simulink model "RADIAL_BOOST"  (R2020b)
settings: Solver=ode4  StartTime=0.0  StopTime=10000  FixedStep=Dt  RelTol=1e-3
values from neighbouring files (symbols this model uses):
  alpha = 0.01    [INPUTS_GRUPPO20.m]
  dt_RB = m_c0_RB*(dv_RB)/F_thr    [INPUTS_GRUPPO20.m]
  e_ss = 0.02    [INPUTS_GRUPPO20.m]
  enable_drag = 1    [INPUTS_GRUPPO20.m]
  enable_J2 = 1    [INPUTS_GRUPPO20.m]
  enable_Mgrav = 1    [INPUTS_GRUPPO20.m]
  enable_PD = 1    [INPUTS_GRUPPO20.m]
  enable_SMC = 0    [INPUTS_GRUPPO20.m]
  F_D = -1/2*rho*CD*A*Vx^2    (= -3.88125057814e-05)    [INPUTS_GRUPPO20.m]
  F_thr = n*Tmax    (= 2)    [INPUTS_GRUPPO20.m]
  FJ2 = -3*J2*m_c0*mu*r_E^2/(2*r^4)    (= -0.00149705073945)    [INPUTS_GRUPPO20.m]
  gmax = 0.005    [INPUTS_GRUPPO20.m]
  INV_ZZZ = pinv(ZZZ)    [INPUTS_GRUPPO20.m]
  invJ = inv(J)    [INPUTS_GRUPPO20.m]
  Isp1 = 220    [INPUTS_GRUPPO20.m]
  J = J0    [INPUTS_GRUPPO20.m]
  kd = d*eye(3)    [INPUTS_GRUPPO20.m]
  kf = U_max/edb    (= 10)    [INPUTS_GRUPPO20.m]
  kp1 = k*eye(3)    [INPUTS_GRUPPO20.m]
  Kr = 1    [INPUTS_GRUPPO20.m]
  lambda = 0.03    [INPUTS_GRUPPO20.m]
  m_c0_RB = m_H(end)    [INPUTS_GRUPPO20.m]
  omega = (mu/r^3)^0.5    (= 0.00113136572666)    [INPUTS_GRUPPO20.m]
  p_RW = 1    [INPUTS_GRUPPO20.m]
  Pos0 = Pos_RB(end,:)'    [INPUTS_GRUPPO20.m]
  q0_0 = Q_RB(end,1)'    [INPUTS_GRUPPO20.m]
  q_des = [1 0 0 0]'    [INPUTS_GRUPPO20.m]
  qv_0 = Q_RB(end,2:4)'    [INPUTS_GRUPPO20.m]
  tau = -deltaton/log((1-(U_on-U_off)/kf))    [INPUTS_GRUPPO20.m]
  tau_RW = 1.5645e-2    (= 0.015645)    [INPUTS_GRUPPO20.m]
  U_max = 2    [INPUTS_GRUPPO20.m]
  U_off = 0.29    [INPUTS_GRUPPO20.m]
  U_on = 1    [INPUTS_GRUPPO20.m]
  Vel0 = Vel_RB(end,:)'    [INPUTS_GRUPPO20.m]
  wb_0 = wb_RB(end,:)'    [INPUTS_GRUPPO20.m]
  ZZZ = [cos(B)    0      -cos(B)    0 ... (first row only)    [INPUTS_GRUPPO20.m]
undefined symbols (not defined in the file or in its folder): DiscIntNeverNeededParam, magnitude
libraries: vrlib x3, aerolibutil x1, sharedtransform x1
settings Model: Creator=andre  LastModifiedBy=andre

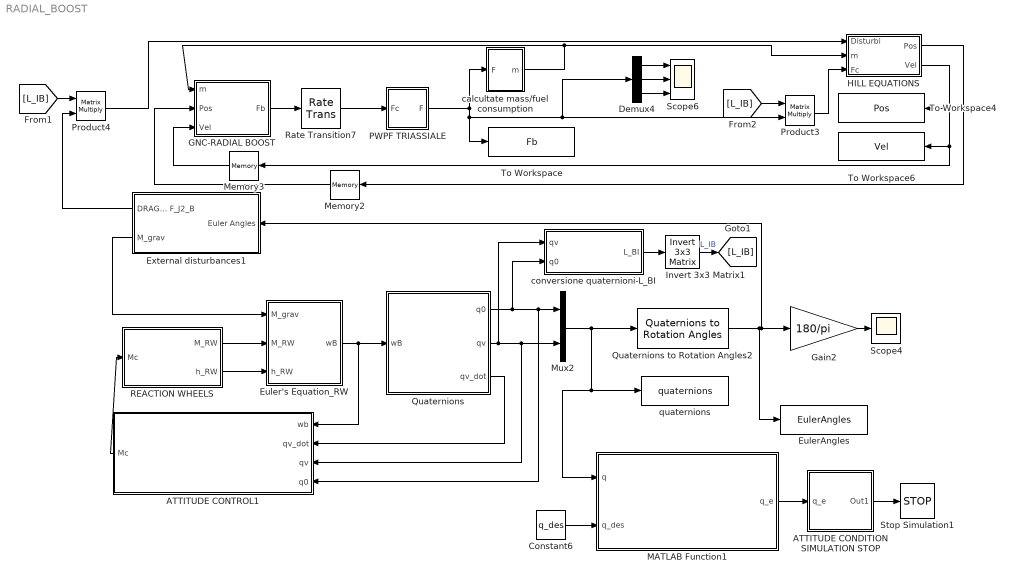
== system RADIAL_BOOST ==
  ATTITUDE CONDITION SIMULATION STOP : Subsystem
  ATTITUDE CONTROL1 : Subsystem
  Constant6 : Constant  Value=q_des
  Demux4 : Demux  Outputs=3
  Euler's Equation_RW : Subsystem
  EulerAngles : ToWorkspace  VariableName=EulerAngles  SampleTime=-1
  External disturbances1 : Subsystem
  GNC-RADIAL BOOST : Subsystem
  Gain2 : Gain  Gain=180/pi
  HILL EQUATIONS : Subsystem
  Invert 3x3 Matrix1 : aerolibutil/Invert  3x3 Matrix
  MATLAB Function1 : MATLAB Function  TreatAsAtomicUnit=on
  Memory2 : Memory  InitialCondition=Pos0
  Memory3 : Memory  InitialCondition=Vel0
  Mux2 : Mux  Inputs=2
  PWPF TRIASSIALE : Subsystem
  Product3 : Product  Multiplication=Matrix(*)
  Product4 : Product  Multiplication=Matrix(*)
  Quaternions : Subsystem
  Quaternions to Rotation Angles2 : sharedtransform/Quaternions to Rotation Angles  rotationOrder=ZYX  aMode=aMode
      settings: SourceProductBaseCode=AE,PW,MT,UV,VE,VP
  REACTION WHEELS : Subsystem
  Rate Transition7 : RateTransition  OutPortSampleTime=Dt
  Scope4 : Scope
  Scope6 : Scope  NumInputPorts=3
  Stop Simulation1 : Stop
  To Workspace : ToWorkspace  VariableName=Fb  SampleTime=-1
  To Workspace4 : ToWorkspace  VariableName=Pos  SampleTime=-1
      settings: Save2DSignal=2-D array (concatenate along first dimension)
  To Workspace6 : ToWorkspace  VariableName=Vel  SampleTime=-1
      settings: Save2DSignal=2-D array (concatenate along first dimension)
  calcultate mass/fuel consumption : Subsystem
  conversione quaternioni-L_BI : Subsystem
  quaternions : ToWorkspace  VariableName=quaternions  SampleTime=-1
  wires:
  Demux4/1 -> Scope6/1
  calcultate mass/fuel consumption/1(m) -> GNC-RADIAL BOOST/1(m), HILL EQUATIONS/2(m)
  [L_IB] -> Product3/1
  conversione quaternioni-L_BI/1(L_BI) -> Invert 3x3 Matrix1/1
  Memory3/1 -> GNC-RADIAL BOOST/3(Vel)
  Gain2/1 -> Scope4/1
  External disturbances1/2(M_grav) -> Euler's Equation_RW/1(M_grav)
  Quaternions/3(qv_dot) -> ATTITUDE CONTROL1/2(qv_dot)
  GNC-RADIAL BOOST/1(Fb) -> Rate Transition7/1
  Rate Transition7/1 -> PWPF TRIASSIALE/1(Fc)
  Quaternions to Rotation Angles2/1 -> Gain2/1, External disturbances1/1(Euler Angles), EulerAngles/1
  [L_IB] -> Product4/1
  HILL EQUATIONS/2(Vel) -> Memory3/1, To Workspace6/1
  PWPF TRIASSIALE/1(F) -> Demux4/1, Product3/2, To Workspace/1, calcultate mass/fuel consumption/1(F)
  REACTION WHEELS/2("h_RW ") -> Euler's Equation_RW/3(h_RW)
  Invert 3x3 Matrix1/1 -> [L_IB]  "L_IB"
  Demux4/3 -> Scope6/3
  Product3/1 -> HILL EQUATIONS/3(Fc)
  Product4/1 -> HILL EQUATIONS/1(Disturbi)
  Memory2/1 -> GNC-RADIAL BOOST/2(Pos)
  Quaternions/1(q0) -> ATTITUDE CONTROL1/4(q0), Mux2/1, conversione quaternioni-L_BI/2(q0)
  Constant6/1 -> MATLAB Function1/2(q_des)
  REACTION WHEELS/1(M_RW) -> Euler's Equation_RW/2(M_RW)
  Euler's Equation_RW/1(wB) -> ATTITUDE CONTROL1/1(wb), Quaternions/1(wB)
  Demux4/2 -> Scope6/2
  Quaternions/2(qv) -> ATTITUDE CONTROL1/3(qv), Mux2/2, conversione quaternioni-L_BI/1(qv)
  Mux2/1 -> Quaternions to Rotation Angles2/1, quaternions/1, MATLAB Function1/1(q)
  ATTITUDE CONTROL1/1(Mc) -> REACTION WHEELS/1(Mc)
  External disturbances1/1(DRAG_B + F_J2_B) -> Product4/2
  HILL EQUATIONS/1(Pos) -> Memory2/1, To Workspace4/1
  MATLAB Function1/1(q_e) -> ATTITUDE CONDITION SIMULATION STOP/1(q_e)
  ATTITUDE CONDITION SIMULATION STOP/1(Out1) -> Stop Simulation1/1

== system RADIAL_BOOST/ATTITUDE CONDITION SIMULATION STOP ==
  q_e : Inport
  Constant5 : Constant
  Constant7 : Constant  Value=0
  Dot Product2 : DotProduct  InputSameDT=on  OutDataTypeStr=Inherit: Inherit via internal rule
  Square Root2 : Sqrt  SaturateOnIntegerOverflow=on
  Subsystem1 : Subsystem
  Switch1 : Switch  Criteria=u2 > Threshold  Threshold=e_ss
  quaternions1 : ToWorkspace  VariableName=normqerr  SampleTime=-1
  Out1 : Outport
  wires:
  Dot Product2/1 -> Square Root2/1
  Subsystem1/1(q_v_err) -> Dot Product2/1, Dot Product2/2
  Constant7/1 -> Switch1/3
  Square Root2/1 -> quaternions1/1, Switch1/2
  Switch1/1 -> Out1/1
  q_e/1 -> Subsystem1/1(q_e)
  Constant5/1 -> Switch1/1

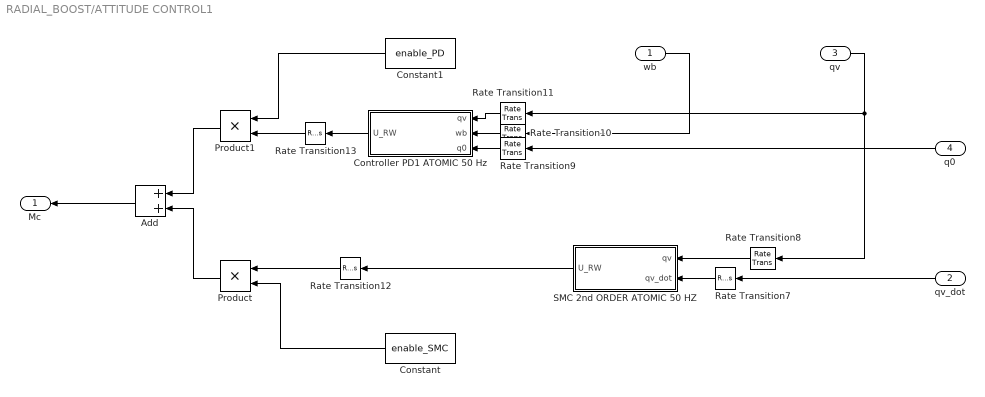
== system RADIAL_BOOST/ATTITUDE CONTROL1 ==
  wb : Inport
  qv_dot : Inport  Port=2
  qv : Inport  Port=3
  q0 : Inport  Port=4
  Add : Sum
  Constant : Constant  Value=enable_SMC
  Constant1 : Constant  Value=enable_PD
  Controller PD1 ATOMIC 50 Hz : Subsystem  TreatAsAtomicUnit=on  SystemSampleTime=0.02
  Product : Product
  Product1 : Product
  Rate Transition10 : RateTransition  InitialCondition=wb_0  OutPortSampleTime=Dt_con
  Rate Transition11 : RateTransition  InitialCondition=qv_0  OutPortSampleTime=Dt_con
  Rate Transition12 : RateTransition  OutPortSampleTime=Dt
  Rate Transition13 : RateTransition  OutPortSampleTime=Dt
  Rate Transition7 : RateTransition  InitialCondition=qv_0  OutPortSampleTime=Dt_con
  Rate Transition8 : RateTransition  InitialCondition=q0_0  OutPortSampleTime=Dt_con
  Rate Transition9 : RateTransition  InitialCondition=q0_0  OutPortSampleTime=Dt_con
  SMC 2nd ORDER ATOMIC 50 HZ : Subsystem  TreatAsAtomicUnit=on  SystemSampleTime=0.02
  Mc : Outport
  wires:
  Add/1 -> Mc/1
  qv_dot/1 -> Rate Transition7/1
  q0/1 -> Rate Transition9/1
  SMC 2nd ORDER ATOMIC 50 HZ/1(U_RW) -> Rate Transition12/1
  Controller PD1 ATOMIC 50 Hz/1(U_RW) -> Rate Transition13/1
  Rate Transition8/1 -> SMC 2nd ORDER ATOMIC 50 HZ/1(qv)
  wb/1 -> Rate Transition10/1
  Rate Transition7/1 -> SMC 2nd ORDER ATOMIC 50 HZ/2(qv_dot)
  Rate Transition10/1 -> Controller PD1 ATOMIC 50 Hz/2(wb)
  Rate Transition11/1 -> Controller PD1 ATOMIC 50 Hz/1(qv)
  qv/1 -> Rate Transition11/1, Rate Transition8/1
  Rate Transition9/1 -> Controller PD1 ATOMIC 50 Hz/3(q0)
  Rate Transition12/1 -> Product/1
  Constant/1 -> Product/2
  Rate Transition13/1 -> Product1/2
  Constant1/1 -> Product1/1
  Product1/1 -> Add/1
  Product/1 -> Add/2

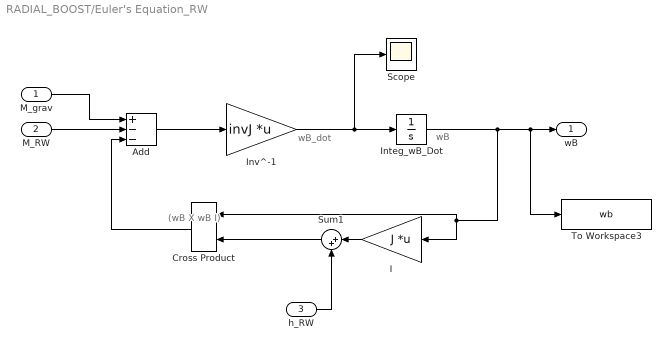
== system RADIAL_BOOST/Euler's Equation_RW ==
  note: (wB X wB I)
  note: wB
  note: wB_dot
  M_grav : Inport
  M_RW : Inport  Port=2
  h_RW : Inport  Port=3
  Add : Sum  Inputs=+--
  Cross Product : vrlib/Utilities/Cross Product
  I : Gain  Gain=J  Multiplication=Matrix(K*u)
  Integ_wB_Dot : Integrator  InitialCondition=wb_0
  Inv^-1 : Gain  Gain=invJ  Multiplication=Matrix(K*u)
  Scope : Scope
  Sum1 : Sum  Inputs=|++
  To Workspace3 : ToWorkspace  VariableName=wb  SampleTime=-1
  wB : Outport  VectorParamsAs1DForOutWhenUnconnected=off
  wires:
  M_grav/1 -> Add/1
  Sum1/1 -> Cross Product/2
  h_RW/1 -> Sum1/2
  Integ_wB_Dot/1 -> To Workspace3/1, wB/1, Cross Product/1, I/1
  I/1 -> Sum1/1
  M_RW/1 -> Add/2
  Add/1 -> Inv^-1/1
  Inv^-1/1 -> Scope/1, Integ_wB_Dot/1
  Cross Product/1 -> Add/3

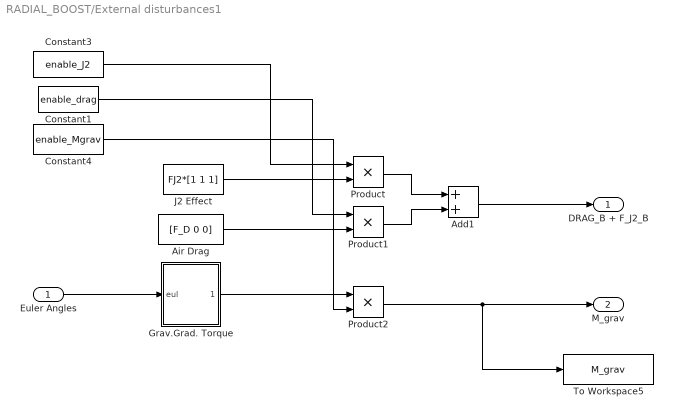
== system RADIAL_BOOST/External disturbances1 ==
  Euler Angles : Inport
  Add1 : Sum
  Air Drag : Constant  Value=[F_D 0 0]
  Constant1 : Constant  Value=enable_drag
  Constant3 : Constant  Value=enable_J2
  Constant4 : Constant  Value=enable_Mgrav
  Grav.Grad. Torque : Subsystem
  J2 Effect : Constant  Value=FJ2*[1 1 1]
  Product : Product
  Product1 : Product
  Product2 : Product
  To Workspace5 : ToWorkspace  VariableName=M_grav  SampleTime=-1
  DRAG_B + F_J2_B : Outport
  M_grav : Outport  Port=2
  wires:
  Grav.Grad. Torque/1(M_grav) -> Product2/1
  Euler Angles/1 -> Grav.Grad. Torque/1(eul)
  Add1/1 -> DRAG_B + F_J2_B/1
  Constant3/1 -> Product/1
  J2 Effect/1 -> Product/2
  Constant1/1 -> Product1/1
  Air Drag/1 -> Product1/2
  Constant4/1 -> Product2/2
  Product/1 -> Add1/1
  Product1/1 -> Add1/2
  Product2/1 -> To Workspace5/1, M_grav/1

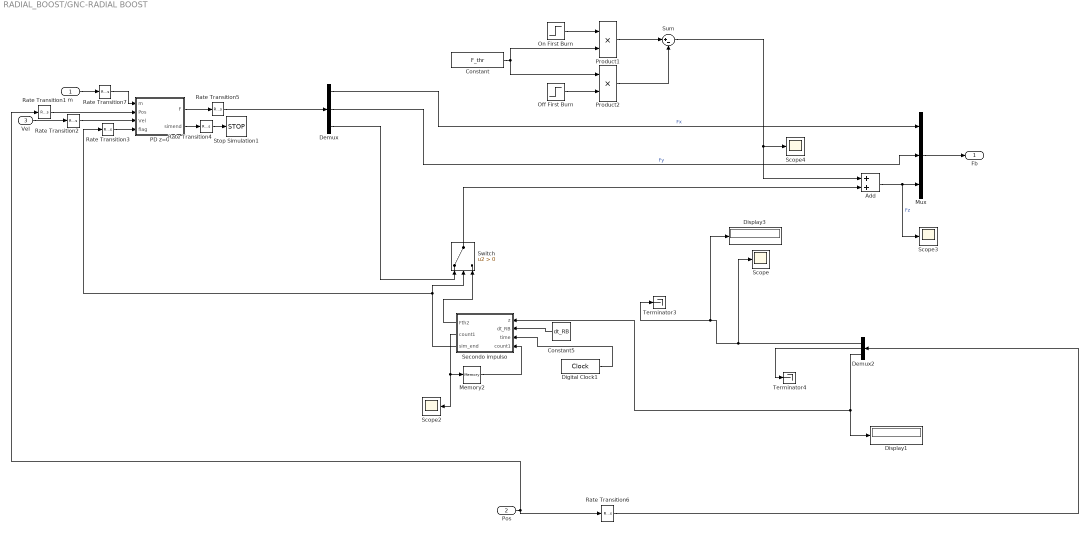
== system RADIAL_BOOST/GNC-RADIAL BOOST ==
  m : Inport
  Pos : Inport  Port=2
  Vel : Inport  Port=3
  Add : Sum
  Constant : Constant  Value=F_thr
  Constant5 : Constant  Value=dt_RB
  Demux : Demux  Outputs=3
  Demux2 : Demux  Outputs=3
  Digital Clock1 : DigitalClock
  Display1 : Display
  Display3 : Display
  Memory2 : Memory  InheritSampleTime=on
  Mux : Mux  Inputs=3
  Off First Burn : Step  Time=dt_RB  After=+1  SampleTime=1
  On First Burn : Step  Time=0  SampleTime=1
  PD z=0 : MATLAB Function  TreatAsAtomicUnit=on
  Product1 : Product
  Product2 : Product
  Rate Transition1 : RateTransition  InitialCondition=Pos0  OutPortSampleTime=Dt_con
  Rate Transition2 : RateTransition  InitialCondition=Vel0  OutPortSampleTime=Dt_con
  Rate Transition3 : RateTransition  OutPortSampleTime=Dt_con
  Rate Transition4 : RateTransition  OutPortSampleTime=Dt_guid
  Rate Transition5 : RateTransition  OutPortSampleTime=Dt_guid
  Rate Transition6 : RateTransition  InitialCondition=Pos0  OutPortSampleTime=Dt_guid
  Rate Transition7 : RateTransition  InitialCondition=m_c0_RB  OutPortSampleTime=Dt_con
  Scope{,2..4} (4 alike) : Scope
  Secondo impulso : MATLAB Function  TreatAsAtomicUnit=on
  Stop Simulation1 : Stop
  Sum : Sum  Inputs=|+-
  Switch : Switch  Criteria=u2 > Threshold
  Terminator3 : Terminator
  Terminator4 : Terminator
  Fb : Outport
  wires:
  Rate Transition7/1 -> PD z=0/1(m)
  Vel/1 -> Rate Transition2/1
  Switch/1 -> Add/2
  Rate Transition3/1 -> PD z=0/4(flag)
  Rate Transition1/1 -> PD z=0/2(Pos)
  PD z=0/2(simend) -> Rate Transition4/1
  Sum/1 -> Add/1, Scope4/1
  Constant5/1 -> Secondo impulso/2(dt_RB)
  Secondo impulso/3(sim_end) -> Rate Transition3/1, Switch/2
  Secondo impulso/2(count1) -> Memory2/1, Scope2/1
  Product1/1 -> Sum/1
  Demux/2 -> Mux/2  "Fy"
  Product2/1 -> Sum/2
  Off First Burn/1 -> Product2/2
  Digital Clock1/1 -> Secondo impulso/3(time)
  Demux2/2 -> Terminator4/1
  Pos/1 -> Rate Transition1/1, Rate Transition6/1
  Constant/1 -> Product2/1, Product1/2
  Add/1 -> Mux/3, Scope3/1  "Fz"
  Demux2/3 -> Secondo impulso/1(z), Display1/1
  Rate Transition2/1 -> PD z=0/3(Vel)
  On First Burn/1 -> Product1/1
  Demux2/1 -> Display3/1, Terminator3/1, Scope/1
  Secondo impulso/1(Fth2) -> Switch/3
  PD z=0/1(F) -> Rate Transition5/1
  Demux/3 -> Switch/1
  Mux/1 -> Fb/1
  Demux/1 -> Mux/1  "Fx"
  Rate Transition5/1 -> Demux/1
  m/1 -> Rate Transition7/1
  Memory2/1 -> Secondo impulso/4("count1 ")
  Rate Transition4/1 -> Stop Simulation1/1
  Rate Transition6/1 -> Demux2/1

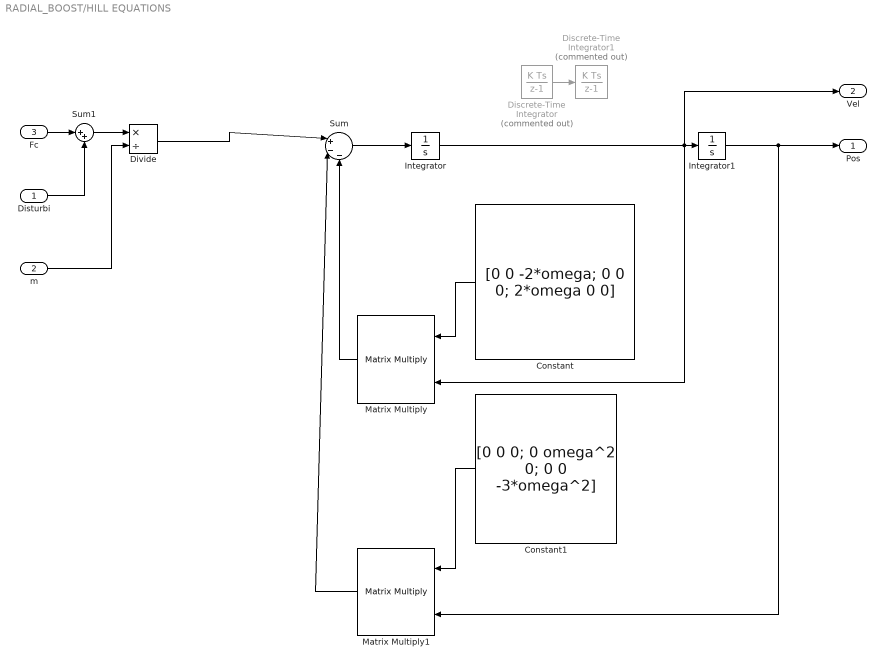
== system RADIAL_BOOST/HILL EQUATIONS ==
  Disturbi : Inport
  m : Inport  Port=2
  Fc : Inport  Port=3
  Constant : Constant  Value=[0 0 -2*omega; 0 0 0; 2*omega 0 0]
  Constant1 : Constant  Value=[0 0 0; 0 omega^2 0; 0 0 -3*omega^2]
  Discrete-Time Integrator : DiscreteIntegrator  Commented=on  InitialCondition=Vel0  SampleTime=-1  ICPrevOutput=DiscIntNeverNeededParam  ICPrevScaledInput=DiscIntNeverNeededParam
  Discrete-Time Integrator1 : DiscreteIntegrator  Commented=on  InitialCondition=Pos0  SampleTime=-1  ICPrevOutput=DiscIntNeverNeededParam  ICPrevScaledInput=DiscIntNeverNeededParam
  Divide : Product  Inputs=*/
  Integrator : Integrator  InitialCondition=Vel0
  Integrator1 : Integrator  InitialCondition=Pos0
  Matrix Multiply : Product  Multiplication=Matrix(*)
  Matrix Multiply1 : Product  Multiplication=Matrix(*)
  Sum : Sum  Inputs=|+--
  Sum1 : Sum  Inputs=|++
  Pos : Outport
  Vel : Outport  Port=2
  wires:
  Constant/1 -> Matrix Multiply/1
  Sum1/1 -> Divide/1
  Disturbi/1 -> Sum1/2
  Integrator/1 -> Integrator1/1, Vel/1, Matrix Multiply/2
  Fc/1 -> Sum1/1
  m/1 -> Divide/2
  Matrix Multiply1/1 -> Sum/2
  Matrix Multiply/1 -> Sum/3
  Constant1/1 -> Matrix Multiply1/1
  Integrator1/1 -> Matrix Multiply1/2, Pos/1
  Sum/1 -> Integrator/1
  Divide/1 -> Sum/1
  Discrete-Time Integrator/1 -> Discrete-Time Integrator1/1

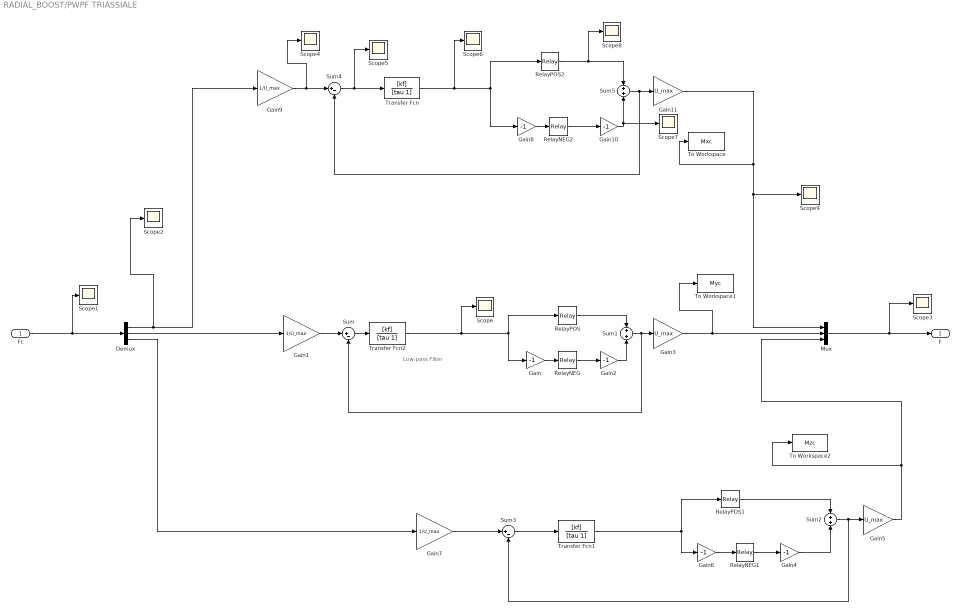
== system RADIAL_BOOST/PWPF TRIASSIALE ==
  note: Low-pass Filter
  Fc : Inport
  Demux : Demux  Outputs=3
  Gain{,2,4,6,8,10} (6 alike) : Gain  Gain=-1
  Gain1 : Gain  Gain=1/U_max
  Gain11 : Gain  Gain=U_max
  Gain3 : Gain  Gain=U_max
  Gain5 : Gain  Gain=U_max
  Gain7 : Gain  Gain=1/U_max
  Gain9 : Gain  Gain=1/U_max
  Mux : Mux  Inputs=3
  RelayNEG : Relay  OnSwitchValue=U_on  OffSwitchValue=U_off
  RelayNEG1 : Relay  OnSwitchValue=U_on  OffSwitchValue=U_off
  RelayNEG2 : Relay  OnSwitchValue=U_on  OffSwitchValue=U_off
  RelayPOS : Relay  OnSwitchValue=U_on  OffSwitchValue=U_off
  RelayPOS1 : Relay  OnSwitchValue=U_on  OffSwitchValue=U_off
  RelayPOS2 : Relay  OnSwitchValue=U_on  OffSwitchValue=U_off
  Scope{,1..9} (10 alike) : Scope
  Sum : Sum  Inputs=|+-
  Sum1 : Sum  Inputs=+|+
  Sum2 : Sum  Inputs=+|+
  Sum3 : Sum  Inputs=|+-
  Sum4 : Sum  Inputs=|+-
  Sum5 : Sum  Inputs=+|+
  To Workspace : ToWorkspace  VariableName=Mxc  SampleTime=-1
  To Workspace1 : ToWorkspace  VariableName=Myc  SampleTime=-1
  To Workspace2 : ToWorkspace  VariableName=Mzc  SampleTime=-1
  Transfer Fcn : TransferFcn  Numerator=[kf]  Denominator=[tau 1]
  Transfer Fcn1 : TransferFcn  Numerator=[kf]  Denominator=[tau 1]
  Transfer Fcn2 : TransferFcn  Numerator=[kf]  Denominator=[tau 1]
  F : Outport  VectorParamsAs1DForOutWhenUnconnected=off
  wires:
  Gain3/1 -> Mux/2, To Workspace1/1
  Gain11/1 -> Scope9/1, Mux/1, To Workspace/1
  Mux/1 -> F/1, Scope3/1
  Gain5/1 -> To Workspace2/1, Mux/3
  Sum5/1 -> Gain11/1, Sum4/2
  RelayPOS2/1 -> Sum5/1, Scope8/1
  Gain10/1 -> Scope7/1, Sum5/2
  Transfer Fcn/1 -> RelayPOS2/1, Gain8/1, Scope6/1
  Gain8/1 -> RelayNEG2/1
  RelayNEG2/1 -> Gain10/1
  Sum4/1 -> Scope5/1, Transfer Fcn/1
  Gain9/1 -> Sum4/1, Scope4/1
  Demux/1 -> Gain9/1, Scope2/1
  Demux/2 -> Gain1/1
  Demux/3 -> Gain7/1
  Gain7/1 -> Sum3/1
  Sum3/1 -> Transfer Fcn1/1
  Sum2/1 -> Gain5/1, Sum3/2
  Gain4/1 -> Sum2/2
  RelayPOS1/1 -> Sum2/1
  RelayNEG1/1 -> Gain4/1
  Gain6/1 -> RelayNEG1/1
  Transfer Fcn1/1 -> RelayPOS1/1, Gain6/1
  Gain2/1 -> Sum1/2
  Sum/1 -> Transfer Fcn2/1
  Gain1/1 -> Sum/1
  Sum1/1 -> Gain3/1, Sum/2
  RelayNEG/1 -> Gain2/1
  RelayPOS/1 -> Sum1/1
  Gain/1 -> RelayNEG/1
  Transfer Fcn2/1 -> Scope/1, RelayPOS/1, Gain/1
  Fc/1 -> Demux/1, Scope1/1

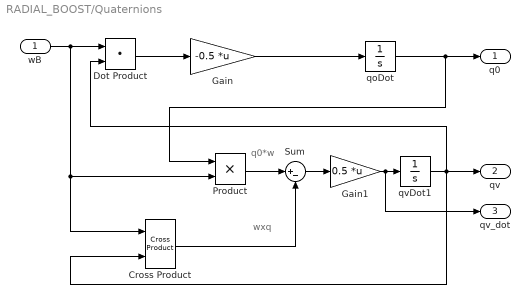
== system RADIAL_BOOST/Quaternions ==
  note: wxq
  note: q0*w
  wB : Inport
  Cross Product : vrlib/Utilities/Cross Product
  Dot Product : DotProduct  InputSameDT=on  OutDataTypeStr=Inherit: Inherit via internal rule
  Gain : Gain  Gain=-0.5  Multiplication=Matrix(K*u)
  Gain1 : Gain  Gain=0.5  Multiplication=Matrix(K*u)
  Product : Product  RndMeth=Zero
  Sum : Sum  Inputs=|+-
  qoDot : Integrator  InitialCondition=q0_0
  qvDot1 : Integrator  InitialCondition=qv_0
  q0 : Outport  VectorParamsAs1DForOutWhenUnconnected=off
  qv : Outport  Port=2  VectorParamsAs1DForOutWhenUnconnected=off
  qv_dot : Outport  Port=3  VectorParamsAs1DForOutWhenUnconnected=off
  wires:
  qoDot/1 -> q0/1, Product/1
  qvDot1/1 -> Cross Product/2, qv/1, Dot Product/2
  wB/1 -> Cross Product/1, Product/2, Dot Product/1
  Dot Product/1 -> Gain/1
  Gain/1 -> qoDot/1
  Product/1 -> Sum/1
  Cross Product/1 -> Sum/2
  Sum/1 -> Gain1/1
  Gain1/1 -> qvDot1/1, qv_dot/1

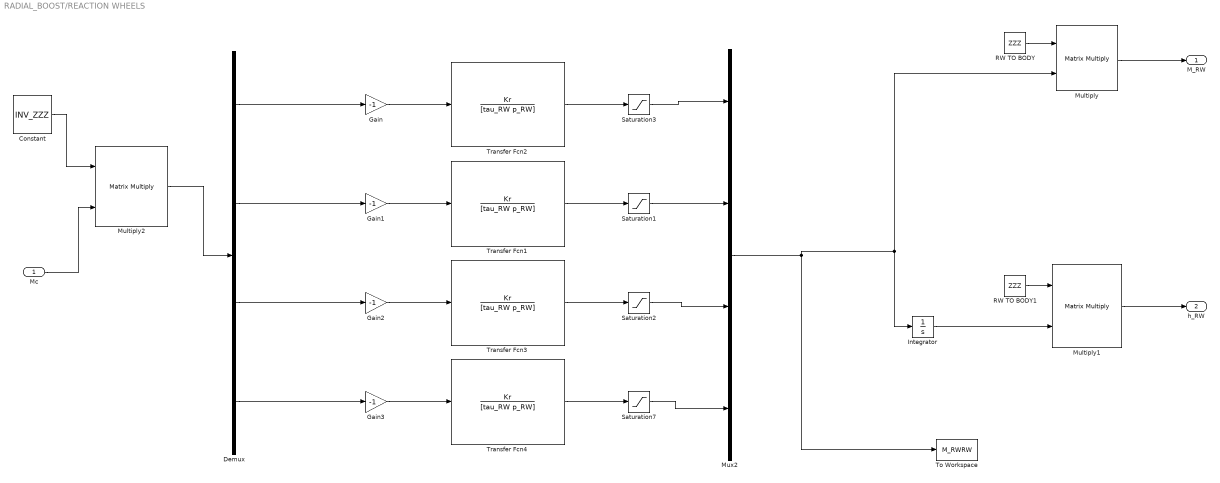
== system RADIAL_BOOST/REACTION WHEELS ==
  Mc : Inport
  Constant : Constant  Value=INV_ZZZ
  Demux : Demux
  Gain{,1..3} (4 alike) : Gain  Gain=-1
  Integrator : Integrator
  Multiply : Product  Multiplication=Matrix(*)
  Multiply1 : Product  Multiplication=Matrix(*)
  Multiply2 : Product  Multiplication=Matrix(*)
  Mux2 : Mux
  RW TO BODY : Constant  Value=ZZZ
  RW TO BODY1 : Constant  Value=ZZZ
  Saturation{1..3,7} (4 alike) : Saturate  UpperLimit=gmax  LowerLimit=-gmax
  To Workspace : ToWorkspace  VariableName=M_RWRW  SampleTime=-1
  Transfer Fcn{1..4} (4 alike) : TransferFcn  Numerator=Kr  Denominator=[tau_RW p_RW]
  M_RW : Outport  VectorParamsAs1DForOutWhenUnconnected=off
  "h_RW " : Outport  Port=2  VectorParamsAs1DForOutWhenUnconnected=off
  wires:
  Mc/1 -> Multiply2/2
  Multiply/1 -> M_RW/1
  Demux/1 -> Gain/1
  Demux/2 -> Gain1/1
  Demux/3 -> Gain2/1
  Gain/1 -> Transfer Fcn2/1
  Gain1/1 -> Transfer Fcn1/1
  Gain2/1 -> Transfer Fcn3/1
  Multiply1/1 -> "h_RW "/1
  Demux/4 -> Gain3/1
  Gain3/1 -> Transfer Fcn4/1
  RW TO BODY/1 -> Multiply/1
  RW TO BODY1/1 -> Multiply1/1
  Constant/1 -> Multiply2/1
  Multiply2/1 -> Demux/1
  Transfer Fcn4/1 -> Saturation7/1
  Mux2/1 -> To Workspace/1, Multiply/2, Integrator/1
  Integrator/1 -> Multiply1/2
  Saturation7/1 -> Mux2/4
  Transfer Fcn3/1 -> Saturation2/1
  Saturation2/1 -> Mux2/3
  Transfer Fcn1/1 -> Saturation1/1
  Saturation1/1 -> Mux2/2
  Transfer Fcn2/1 -> Saturation3/1
  Saturation3/1 -> Mux2/1

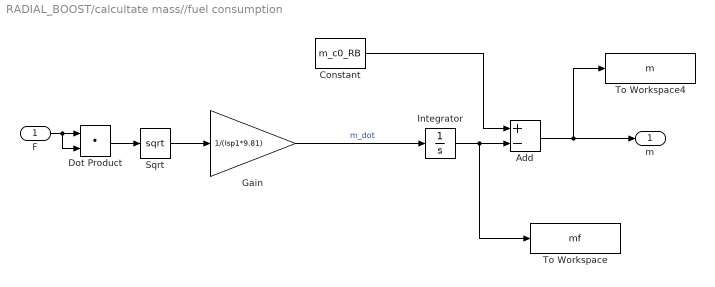
== system RADIAL_BOOST/calcultate mass//fuel consumption ==
  F : Inport
  Add : Sum  Inputs=+-
  Constant : Constant  Value=m_c0_RB
  Dot Product : DotProduct  InputSameDT=on  OutDataTypeStr=Inherit: Inherit via internal rule
  Gain : Gain  Gain=1/(Isp1*9.81)
  Integrator : Integrator
  Sqrt : Sqrt  SaturateOnIntegerOverflow=on
  To Workspace : ToWorkspace  VariableName=mf  SampleTime=-1
  To Workspace4 : ToWorkspace  VariableName=m  SampleTime=-1
  m : Outport
  wires:
  F/1 -> Dot Product/2, Dot Product/1
  Dot Product/1 -> Sqrt/1
  Sqrt/1 -> Gain/1
  Gain/1 -> Integrator/1  "m_dot"
  Integrator/1 -> To Workspace/1, Add/2
  Constant/1 -> Add/1
  Add/1 -> To Workspace4/1, m/1

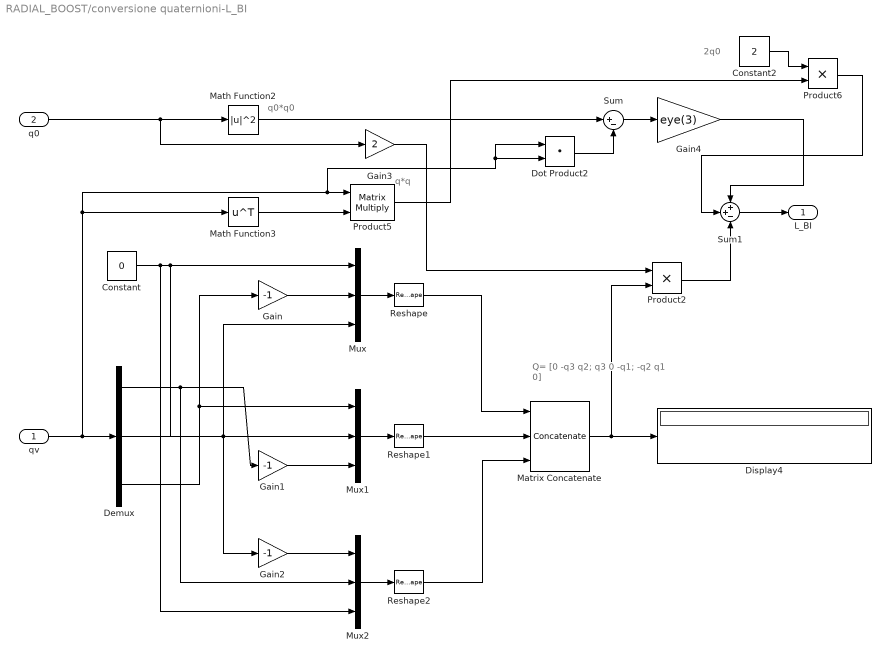
== system RADIAL_BOOST/conversione quaternioni-L_BI ==
  note: Q= [0 -q3 q2;
      | 	q3 0 -q1;
      | 	-q2 q1 0]
  note: 2q0
  note: q*q
  note: q0*q0
  qv : Inport
  q0 : Inport  Port=2
  Constant : Constant  Value=0
  Constant2 : Constant  Value=2
  Demux : Demux  Outputs=3
  Display4 : Display
  Dot Product2 : DotProduct  InputSameDT=on  OutDataTypeStr=Inherit: Inherit via internal rule
  Gain : Gain  Gain=-1
  Gain1 : Gain  Gain=-1
  Gain2 : Gain  Gain=-1
  Gain3 : Gain  Gain=2
  Gain4 : Gain  Gain=eye(3)
  Math Function2 : Math  Operator=magnitude^2  SignedPower=on  SaturateOnIntegerOverflow=on
  Math Function3 : Math  Operator=transpose  SignedPower=on  SaturateOnIntegerOverflow=on
  Matrix Concatenate : Concatenate  NumInputs=3  Mode=Multidimensional array
  Mux : Mux  Inputs=3
  Mux1 : Mux  Inputs=3
  Mux2 : Mux  Inputs=3
  Product2 : Product  RndMeth=Zero
  Product5 : Product  Multiplication=Matrix(*)
  Product6 : Product
  Reshape : Reshape  OutputDimensionality=Row vector (2-D)
  Reshape1 : Reshape  OutputDimensionality=Row vector (2-D)
  Reshape2 : Reshape  OutputDimensionality=Row vector (2-D)
  Sum : Sum  Inputs=|+-
  Sum1 : Sum  Inputs=++-
  L_BI : Outport  VectorParamsAs1DForOutWhenUnconnected=off
  wires:
  qv/1 -> Demux/1, Product5/1, Dot Product2/2, Dot Product2/1, Math Function3/1
  Constant/1 -> Mux/1, Mux1/2, Mux2/3
  Demux/3 -> Gain/1, Mux1/1
  Gain/1 -> Mux/2
  Demux/2 -> Mux/3, Gain2/1
  Gain1/1 -> Mux1/3
  Demux/1 -> Gain1/1, Mux2/2
  Gain2/1 -> Mux2/1
  q0/1 -> Gain3/1, Math Function2/1
  Math Function2/1 -> Sum/1
  Gain4/1 -> Sum1/1
  Product6/1 -> Sum1/2
  Product2/1 -> Sum1/3
  Sum1/1 -> L_BI/1
  Matrix Concatenate/1 -> Product2/2, Display4/1
  Mux/1 -> Reshape/1
  Reshape/1 -> Matrix Concatenate/1
  Mux2/1 -> Reshape2/1
  Reshape2/1 -> Matrix Concatenate/3
  Mux1/1 -> Reshape1/1
  Reshape1/1 -> Matrix Concatenate/2
  Sum/1 -> Gain4/1
  Math Function3/1 -> Product5/2
  Gain3/1 -> Product2/1
  Product5/1 -> Product6/2
  Constant2/1 -> Product6/1
  Dot Product2/1 -> Sum/2

== system RADIAL_BOOST/ATTITUDE CONDITION SIMULATION STOP/Subsystem1 ==
  q_e : Inport
  Demux : Demux
  Mux1 : Mux  Inputs=3
  Terminator : Terminator
  q_v_err : Outport  VectorParamsAs1DForOutWhenUnconnected=off
  wires:
  Demux/3 -> Mux1/2
  Demux/2 -> Mux1/1
  Demux/4 -> Mux1/3
  Demux/1 -> Terminator/1
  q_e/1 -> Demux/1
  Mux1/1 -> q_v_err/1

== system RADIAL_BOOST/ATTITUDE CONTROL1/Controller PD1 ATOMIC 50 Hz ==
  qv : Inport
  wb : Inport  Port=2
  q0 : Inport  Port=3
  Constant : Constant  Value=kp1
  Gain : Gain  Gain=kd  Multiplication=Matrix(K*u) (u vector)
  Multiply : Product  Multiplication=Matrix(*)
  Multiply1 : Product
  Sign : Signum
  Sum : Sum  Inputs=|--
  U_RW : Outport  VectorParamsAs1DForOutWhenUnconnected=off
  wires:
  Gain/1 -> Sum/1
  Constant/1 -> Multiply/1
  q0/1 -> Sign/1
  Multiply/1 -> Multiply1/1
  wb/1 -> Gain/1
  Sign/1 -> Multiply1/2
  Multiply1/1 -> Sum/2
  Sum/1 -> U_RW/1
  qv/1 -> Multiply/2

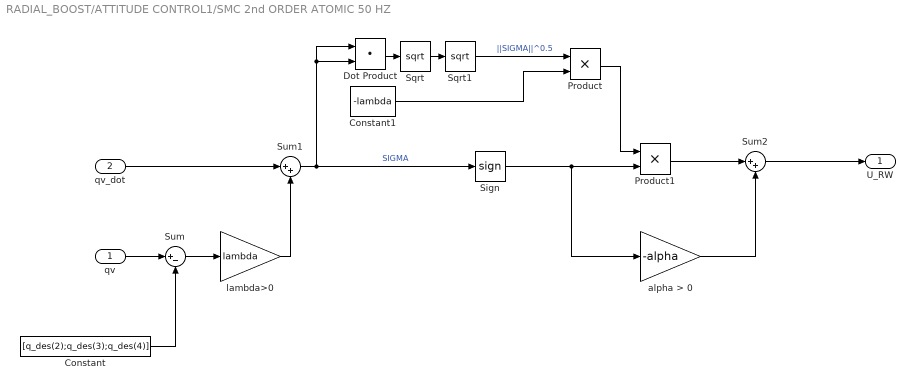
== system RADIAL_BOOST/ATTITUDE CONTROL1/SMC 2nd ORDER ATOMIC 50 HZ ==
  qv : Inport
  qv_dot : Inport  Port=2
  Constant : Constant  Value=[q_des(2);q_des(3);q_des(4)]
  Constant1 : Constant  Value=-lambda
  Dot Product : DotProduct  InputSameDT=on  OutDataTypeStr=Inherit: Inherit via internal rule
  Product : Product
  Product1 : Product
  Sign : Signum
  Sqrt : Sqrt  SaturateOnIntegerOverflow=on
  Sqrt1 : Sqrt  SaturateOnIntegerOverflow=on
  Sum : Sum  Inputs=|+-
  Sum1 : Sum  Inputs=|++
  Sum2 : Sum  Inputs=|++
  alpha > 0 : Gain  Gain=-alpha
  lambda>0 : Gain  Gain=lambda
  U_RW : Outport
  wires:
  Constant1/1 -> Product/2
  alpha > 0/1 -> Sum2/2
  Product1/1 -> Sum2/1
  Dot Product/1 -> Sqrt/1
  Sum/1 -> lambda>0/1
  Sum2/1 -> U_RW/1
  Product/1 -> Product1/1
  Sign/1 -> alpha > 0/1, Product1/2
  lambda>0/1 -> Sum1/2
  Constant/1 -> Sum/2
  Sum1/1 -> Sign/1, Dot Product/1, Dot Product/2  "SIGMA"
  Sqrt/1 -> Sqrt1/1
  Sqrt1/1 -> Product/1  "||SIGMA||^0.5"
  qv_dot/1 -> Sum1/1
  qv/1 -> Sum/1

== system RADIAL_BOOST/External disturbances1/Grav.Grad. Torque ==
  eul : Inport
  Constant3 : Constant  Value=J
  Constant4 : Constant  Value=3*omega^2
  Cross Product : vrlib/Utilities/Cross Product
  MATLAB function : MATLAB Function  TreatAsAtomicUnit=on
  Matrix Multiply : Product  Multiplication=Matrix(*)
  Product2 : Product
  M_grav : Outport
  wires:
  Constant3/1 -> Matrix Multiply/1
  MATLAB function/1(r) -> Matrix Multiply/2, Cross Product/1
  Cross Product/1 -> Product2/2
  Constant4/1 -> Product2/1
  Product2/1 -> M_grav/1
  eul/1 -> MATLAB function/1(eul)
  Matrix Multiply/1 -> Cross Product/2

== matlab function RADIAL_BOOST/External disturbances1/Grav.Grad. Torque/MATLAB function ==
  data: eul input; r output
function r = fcn(eul)
    r = [-sin(eul(2)); sin(eul(3)); 1-(sin(eul(2)))^2-(sin(eul(3)))^2];

== matlab function RADIAL_BOOST/GNC-RADIAL BOOST/Secondo impulso ==
  data: z input; Fth2 output; count1 output; dt_RB input; time input; count1 input; sim_end output
function [Fth2,count1,sim_end] = fcn(z,dt_RB,time, count1)
Dt=1;
Fth = 2;
% if flag_H==0
%     Fth2=0;
%     count1=0;
%     %sim_end=0;
% else
% if x>-500&&time>dt_RB*2&&count1*Dt<dt_RB
if z<1&&time>dt_RB*2&&count1*Dt<dt_RB
    Fth2=Fth;
    count1=count1+1;
    sim_end=0;
%elseif x>=-500&&count1*Dt>dt_RB
elseif count1*Dt>dt_RB
    Fth2=0;
    sim_end=1;
    count1=count1;
elseif count1*Dt>dt_RB
    Fth2=0;
    sim_end=1;
    count1=count1;
else
    count1=count1;
    Fth2=0;
    sim_end=0;
end

== matlab function RADIAL_BOOST/GNC-RADIAL BOOST/PD z=0 ==
  data: m input; F output; Pos input; Vel input; flag input; simend output
function [F,simend]  = fcn(m, Pos,Vel,flag)
simend=0;
F=[0 0 0]';
%m_c0=120;
x_des=[-500 0 0]';
Kp=[0.01 0.01 0.01]';%[0.02 0.01 0.01]';
Kd=0.5;
xdot_des=[0 0 0]';
% if Pos(3)<=50
%     Kp=0.0001;
%     Kd=1;
% end
if flag==1
    xdot=(xdot_des-Vel)*Kd+(x_des-Pos).*Kp;
    F=xdot*m;
end
if Pos(3)<0.5&&Pos(3)>-0.5&&Pos(2)<0.5&&Pos(2)>-0.5&&flag==1
    simend=1;
end
%F(2)=0;

== matlab function RADIAL_BOOST/MATLAB Function1 ==
  data: q input; q_e output; q_des input
function q_e = quaternion_error(q, q_des)
%#codegen

q_inv = [q_des(1) -q_des(2) -q_des(3) -q_des(4)]'/(q_des(1)^2+q_des(2)^2 + q_des(3)^2+q_des(4)^2);

Q   = [q_inv(1) -q_inv(2) -q_inv(3) -q_inv(4)
       q_inv(2)  q_inv(1) -q_inv(4)  q_inv(3)
       q_inv(3)  q_inv(4)  q_inv(1) -q_inv(2)
       q_inv(4) -q_inv(3)  q_inv(2)  q_inv(1)];
q_e =Q*q;
